simulink model "tp412721"  (Simulink 3.0)
settings: Solver=ode1  SolverMode=SingleTasking  StartTime=0.0  StopTime=t_sim  FixedStep=Ts  RelTol=1e-3
values from neighbouring files (symbols this model uses):
  D = exp(-a*Ts)    [init_bulb_fan_PI1_disc_windupless.m]
  P = KR    [init_bulb_fan_PI1_disc_windupless.m]
  Ts = 1    [init_bulb_fan_PI1_disc_windupless.m]    (also in prev45_10.mat = 0.2; prev45_2.mat = 0.2; prev45_4.mat = 0.2)
  Umax = 5    [init_bulb_fan_PI1_disc_windupless.m]    (also in prev45_10.mat; prev45_2.mat; prev45_4.mat)
  Umin = -5    [init_bulb_fan_PI1_disc_windupless.m]    (also in prev45_10.mat = 0; prev45_2.mat = 0; prev45_4.mat = 0)
undefined symbols (not defined in the file or in its folder): I
libraries: udaq28LT_lib x1
settings Model: LastModifiedBy=mato  SaveFormat=Matrix  BooleanDataType=on

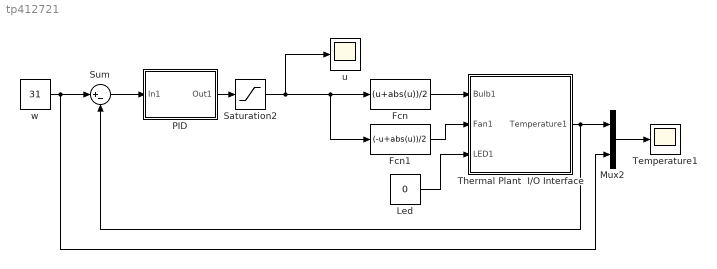
== system tp412721 ==
  Fcn : Fcn  Expr=(u+abs(u))/2
  Fcn1 : Fcn  Expr=(-u+abs(u))/2
  Led : Constant  Value=0
  Mux2 : Mux  Inputs=2
  PID : Subsystem
  Saturation2 : Saturate  UpperLimit=Umax  LowerLimit=Umin
  Sum : Sum  Inputs=|+-  SaturateOnIntegerOverflow=on
  Temperature1 : Scope
      settings: TickLabels=on  TimeRange=30  YMin=15  YMax=50  SaveName=yt  DataFormat=Matrix
  Thermal Plant  I/O Interface : Subsystem
      mask Display: disp('Thermo-optical\nPlant\nI/O Interface')
  u : Scope
      settings: TimeRange=120  YMin=-0.5  YMax=5.5  SaveName=u  DataFormat=Matrix  Decimation=10  SampleInput=on  SampleTime=Ts
  w : Constant  Value=31
  wires:
  Sum/1 -> PID/1(In1)
  PID/1(Out1) -> Saturation2/1
  w/1 -> Sum/1, Mux2/2
  Mux2/1 -> Temperature1/1
  Saturation2/1 -> u/1, Fcn/1, Fcn1/1
  Fcn/1 -> Thermal Plant  I/O Interface/1(Bulb1)
  Fcn1/1 -> Thermal Plant  I/O Interface/2(Fan1)
  Led/1 -> Thermal Plant  I/O Interface/3(LED1)
  Thermal Plant  I/O Interface/1(Temperature1) -> Mux2/1, Sum/2

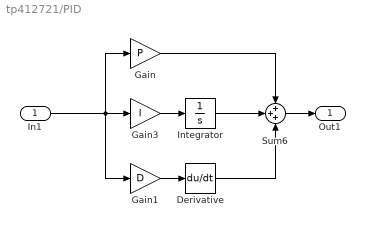
== system tp412721/PID ==
  In1 : Inport  Port=1  PortWidth=-1  SampleTime=-1  DataType=auto
      settings: SignalType=auto
  Derivative : Derivative
  Gain : Gain  Gain=P  SaturateOnIntegerOverflow=on
  Gain1 : Gain  Gain=D  SaturateOnIntegerOverflow=on
  Gain3 : Gain  Gain=I  SaturateOnIntegerOverflow=on
  Integrator : Integrator  ExternalReset=none  InitialConditionSource=internal  InitialCondition=0  LimitOutput=off  UpperSaturationLimit=inf  LowerSaturationLimit=-inf  ShowSaturationPort=off  ShowStatePort=off  AbsoluteTolerance=auto
  Sum6 : Sum  Inputs=+++  SaturateOnIntegerOverflow=on
  Out1 : Outport  Port=1
  wires:
  Gain3/1 -> Integrator/1
  Sum6/1 -> Out1/1
  In1/1 -> Gain/1, Gain3/1, Gain1/1
  Integrator/1 -> Sum6/2
  Gain/1 -> Sum6/1
  Gain1/1 -> Derivative/1
  Derivative/1 -> Sum6/3

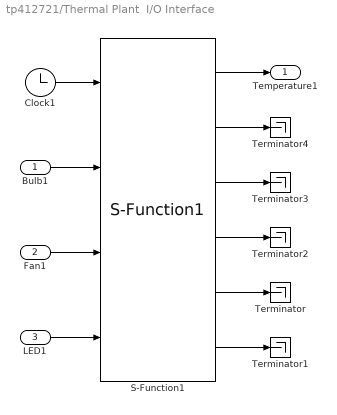
== system tp412721/Thermal Plant  I/O Interface ==
  Bulb1 : Inport  Port=1  PortWidth=-1  SampleTime=-1  DataType=auto
      settings: SignalType=auto
  Fan1 : Inport  Port=2  PortWidth=-1  SampleTime=-1  DataType=auto
      settings: SignalType=auto
  LED1 : Inport  Port=3  PortWidth=-1  SampleTime=-1  DataType=auto
      settings: SignalType=auto
  Clock1 : Clock
      settings: DisplayTime=off  Decimation=10
  S-Function1 : udaq28LT_lib/S-Function1  Priority=1  com_port=COM3  Ts=Ts  events_ot=2  rd_timeout=Ts/2*1000  matlab_prior=ABOVE_NORMAL_PRIORITY  warning=on  printout=off
  Terminator{,1..4} (5 alike) : Terminator
  Temperature1 : Outport  Port=1
  wires:
  S-Function1/1 -> Temperature1/1
  S-Function1/2 -> Terminator4/1
  Clock1/1 -> S-Function1/1
  Bulb1/1 -> S-Function1/2
  Fan1/1 -> S-Function1/3
  S-Function1/3 -> Terminator3/1
  S-Function1/4 -> Terminator2/1
  S-Function1/5 -> Terminator/1
  S-Function1/6 -> Terminator1/1
  LED1/1 -> S-Function1/4
